simulink model "remoteMicrogrid"  (R2023a)
settings: Solver=FixedStepDiscrete  StartTime=0.0  StopTime=8  FixedStep=Ts  RelTol=1e-3
PreLoadFcn:
  | remoteMicrogridInputData
undefined symbols (not defined in the file): BESS, ControlRoom, DiscIntNeverNeededParam, Grid, Load, Machine, Microgrid, PV, T_on, Ts
libraries: ee_lib x46, eeGeneralControl x35, nesl_utility_internal x25, simulink x24, nesl_utility x20, fl_lib x17, slpidlib x12, eeTransforms x5, eeRmsMeasurement x4, eeTotalHarmonicDistorsion x4, eeSinusoidalMeasurement x3, batteryecm_lib x2
(part 4 of 5)

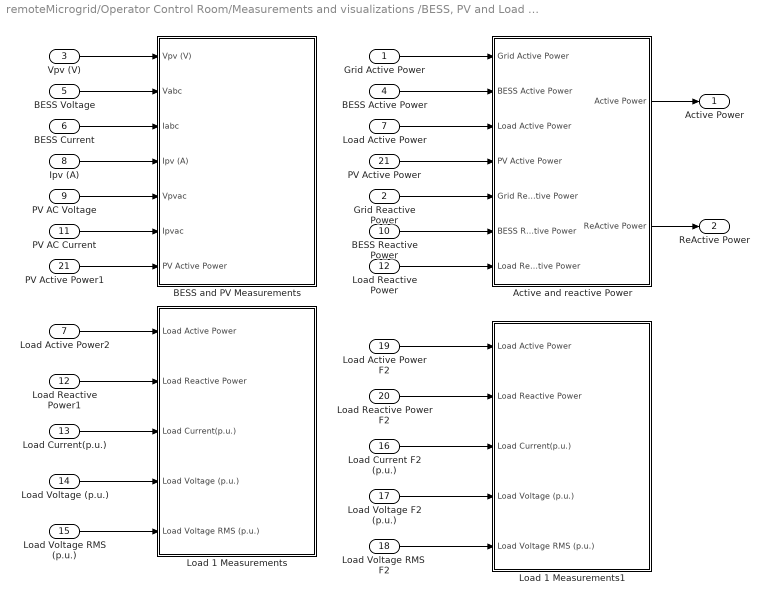
== system remoteMicrogrid/Operator Control Room/Measurements and visualizations /BESS, PV and Load Measurements ==
  Grid Active Power : Inport
  Grid Reactive Power : Inport  Port=2
  Vpv (V) : Inport  Port=3
  BESS Active Power : Inport  Port=4
  BESS Voltage : Inport  Port=5
  BESS Current : Inport  Port=6
  Load Active Power : Inport  Port=7
  Ipv (A) : Inport  Port=8
  PV AC Voltage : Inport  Port=9
  BESS Reactive Power : Inport  Port=10
  PV AC Current : Inport  Port=11
  Load Reactive Power : Inport  Port=12
  Load Current(p.u.) : Inport  Port=13
  Load Voltage (p.u.) : Inport  Port=14
  Load Voltage RMS (p.u.) : Inport  Port=15
  Load Current F2 (p.u.) : Inport  Port=16
  Load Voltage F2 (p.u.) : Inport  Port=17
  Load Voltage RMS  F2 : Inport  Port=18
  "Load Active Power F2 " : Inport  Port=19
  Load Reactive Power F2 : Inport  Port=20
  PV Active Power : Inport  Port=21
  Active and reactive Power : Subsystem
  BESS and PV Measurements : Subsystem
  Load 1 Measurements : Subsystem
  Load 1 Measurements1 : Subsystem
  Load Active Power2 : InportShadow  Port=7
  Load Reactive Power1 : InportShadow  Port=12
  PV Active Power1 : InportShadow  Port=21
  Active Power : Outport
  ReActive Power : Outport  Port=2
  wires:
  Vpv (V)/1 -> BESS and PV Measurements/1(Vpv (V))
  PV AC Current/1 -> BESS and PV Measurements/6(Ipvac)
  BESS Voltage/1 -> BESS and PV Measurements/2(Vabc)
  Load Reactive Power1/1 -> Load 1 Measurements/2(Load Reactive Power)
  PV AC Voltage/1 -> BESS and PV Measurements/5(Vpvac)
  Ipv (A)/1 -> BESS and PV Measurements/4(Ipv (A))
  BESS Current/1 -> BESS and PV Measurements/3(Iabc)
  BESS Reactive Power/1 -> Active and reactive Power/6(BESS Reactive Power)
  Load Voltage (p.u.)/1 -> Load 1 Measurements/4(Load Voltage (p.u.))
  Load Current(p.u.)/1 -> Load 1 Measurements/3(Load Current(p.u.))
  Load Active Power2/1 -> Load 1 Measurements/1(Load Active Power)
  Load Active Power/1 -> Active and reactive Power/3(Load Active Power)
  Load Voltage RMS (p.u.)/1 -> Load 1 Measurements/5(Load Voltage RMS (p.u.))
  Grid Active Power/1 -> Active and reactive Power/1(Grid Active Power)
  BESS Active Power/1 -> Active and reactive Power/2(BESS Active Power)
  Grid Reactive Power/1 -> Active and reactive Power/5(Grid Reactive Power)
  Load Reactive Power/1 -> Active and reactive Power/7(Load Reactive Power)
  "Load Active Power F2 "/1 -> Load 1 Measurements1/1(Load Active Power)
  Load Reactive Power F2/1 -> Load 1 Measurements1/2(Load Reactive Power)
  Load Current F2 (p.u.)/1 -> Load 1 Measurements1/3(Load Current(p.u.))
  Load Voltage F2 (p.u.)/1 -> Load 1 Measurements1/4(Load Voltage (p.u.))
  Load Voltage RMS  F2/1 -> Load 1 Measurements1/5(Load Voltage RMS (p.u.))
  PV Active Power/1 -> Active and reactive Power/4(PV Active Power)
  PV Active Power1/1 -> BESS and PV Measurements/7(PV Active Power)
  Active and reactive Power/1(Active Power) -> Active Power/1
  Active and reactive Power/2(ReActive Power) -> ReActive Power/1

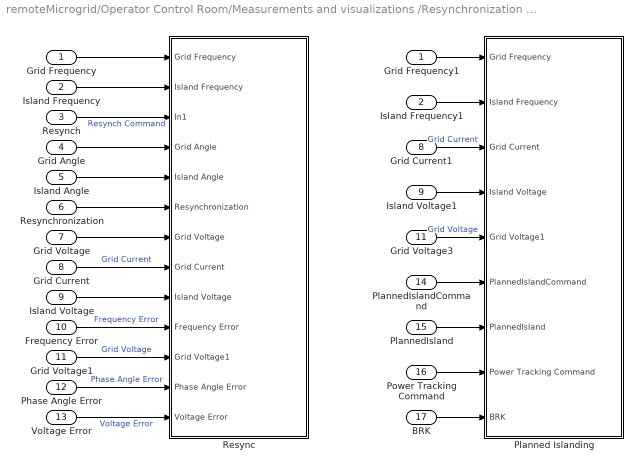
== system remoteMicrogrid/Operator Control Room/Measurements and visualizations /Resynchronization and Planned Islanding ==
  Grid Frequency : Inport
  Island Frequency : Inport  Port=2
  Resynch : Inport  Port=3
  Grid Angle : Inport  Port=4
  Island Angle : Inport  Port=5
  Resynchronization : Inport  Port=6
  Grid Voltage : Inport  Port=7
  Grid Current : Inport  Port=8
  Island Voltage : Inport  Port=9
  Frequency Error : Inport  Port=10
  Grid Voltage1 : Inport  Port=11
  Phase Angle Error : Inport  Port=12
  Voltage Error : Inport  Port=13
  PlannedIslandCommand : Inport  Port=14
  PlannedIsland : Inport  Port=15
  Power Tracking Command : Inport  Port=16
  BRK : Inport  Port=17
  Grid Current1 : InportShadow  Port=8
  Grid Frequency1 : InportShadow
  Grid Voltage3 : InportShadow  Port=11
  Island Frequency1 : InportShadow  Port=2
  Island Voltage1 : InportShadow  Port=9
  Planned Islanding : Subsystem
  Resync : Subsystem
  wires:
  Grid Frequency/1 -> Resync/1(Grid Frequency)
  Island Frequency/1 -> Resync/2(Island Frequency)
  Resynch/1 -> Resync/3(In1)  "Resynch Command"
  Grid Angle/1 -> Resync/4(Grid Angle)
  Island Angle/1 -> Resync/5(Island Angle)
  Resynchronization/1 -> Resync/6(Resynchronization)
  Grid Voltage/1 -> Resync/7(Grid Voltage)
  Grid Current/1 -> Resync/8(Grid Current)  "Grid Current"
  Island Voltage/1 -> Resync/9(Island Voltage)
  Frequency Error/1 -> Resync/10(Frequency Error)  "Frequency Error"
  Grid Voltage1/1 -> Resync/11(Grid Voltage1)  "Grid Voltage"
  Phase Angle Error/1 -> Resync/12(Phase Angle Error)  "Phase Angle Error"
  Voltage Error/1 -> Resync/13(Voltage Error)  "Voltage Error"
  Grid Frequency1/1 -> Planned Islanding/1(Grid Frequency)
  Island Frequency1/1 -> Planned Islanding/2(Island Frequency)
  Grid Current1/1 -> Planned Islanding/3(Grid Current)  "Grid Current"
  Island Voltage1/1 -> Planned Islanding/4(Island Voltage)
  Grid Voltage3/1 -> Planned Islanding/5(Grid Voltage1)  "Grid Voltage"
  PlannedIslandCommand/1 -> Planned Islanding/6(PlannedIslandCommand)
  PlannedIsland/1 -> Planned Islanding/7(PlannedIsland)
  Power Tracking Command/1 -> Planned Islanding/8(Power Tracking Command)
  BRK/1 -> Planned Islanding/9(BRK)

== system remoteMicrogrid/Operator Control Room/Monitoring of system performance/Load  ==
  In1 : Inport
  In2 : Inport  Port=2
  In3 : Inport  Port=3
  Constant1 : Constant  Value=0
  Constant2 : Constant  Value=0
  Constant3 : Constant  Value=0
  Gain : Gain  Gain=1/75
  Load Power and  Current MinMax : Scope  NumInputPorts=4
  Load Voltage MINMAX : Scope  NumInputPorts=4
  MinMax Running Resettable1 : simulink/Math Operations/MinMax Running Resettable  Function=min  vinit=1
  MinMax Running Resettable5 : simulink/Math Operations/MinMax Running Resettable  Function=max  vinit=1
  MinMax Running Resettable6 : simulink/Math Operations/MinMax Running Resettable  Function=min  vinit=0.707
  MinMax Running Resettable7 : simulink/Math Operations/MinMax Running Resettable  Function=max  vinit=0.707
  MinMax Running Resettable8 : simulink/Math Operations/MinMax Running Resettable  Function=min  vinit=0.707
  MinMax Running Resettable9 : simulink/Math Operations/MinMax Running Resettable  Function=max  vinit=0.491
  Subsystem4 : Subsystem
  start at 0.2 s2 : Subsystem
  start at 0.2 s4 : Subsystem
  start at 0.2 s5 : Subsystem
  wires:
  Constant2/1 -> MinMax Running Resettable7/2, MinMax Running Resettable6/2
  Constant1/1 -> MinMax Running Resettable1/2, MinMax Running Resettable5/2
  start at 0.2 s4/1(u) -> MinMax Running Resettable9/1, MinMax Running Resettable8/1
  MinMax Running Resettable7/1 -> Load Voltage MINMAX/4  "Load Voltage Max (pu)"
  Constant3/1 -> MinMax Running Resettable9/2, MinMax Running Resettable8/2
  MinMax Running Resettable8/1 -> Load Power and  Current MinMax/3  "Load Current Min (pu)"
  In1/1 -> start at 0.2 s2/1(In1)
  In2/1 -> start at 0.2 s4/1(In1)
  MinMax Running Resettable5/1 -> Load Power and  Current MinMax/2  "Load Power Max (pu)"
  In3/1 -> start at 0.2 s5/1(In1)
  Subsystem4/1(VoltageLow) -> Load Voltage MINMAX/1  "Load Voltage Crossed Low"
  start at 0.2 s2/1(u) -> MinMax Running Resettable7/1, MinMax Running Resettable6/1, Subsystem4/1(Voltage)
  Gain/1 -> MinMax Running Resettable5/1, MinMax Running Resettable1/1
  MinMax Running Resettable9/1 -> Load Power and  Current MinMax/4  "Load Current Max (pu)"
  start at 0.2 s5/1(u) -> Gain/1
  Subsystem4/2(VoltageHigh) -> Load Voltage MINMAX/2  "Load Voltage Crossed High"
  MinMax Running Resettable6/1 -> Load Voltage MINMAX/3  "Load Voltage Min (pu)"
  MinMax Running Resettable1/1 -> Load Power and  Current MinMax/1  "Load Power Min (pu)"

== system remoteMicrogrid/Operator Control Room/Monitoring of system performance/Microgrid ==
  In1 : Inport
  In2 : Inport  Port=2
  Constant : Constant  Value=0
  Constant4 : Constant  Value=0
  Island Frequency MINMAX : Scope  NumInputPorts=4
  Island Voltage MINMAX : Scope  NumInputPorts=4
  Low-Pass Filter (Discrete or Continuous) : eeGeneralControl/Low-Pass Filter (Discrete or Continuous)  K=1  T=0.04  B=inf  A=-inf  init_option=Inherited from block input  x0=0  Ts=Ts
  Low-Pass Filter (Discrete or Continuous)1 : eeGeneralControl/Low-Pass Filter (Discrete or Continuous)  K=1  T=0.04  B=inf  A=-inf  init_option=Inherited from block input  x0=0  Ts=Ts
  MinMax Running Resettable : simulink/Math Operations/MinMax Running Resettable  Function=max  vinit=Grid.Frequency
  MinMax Running Resettable2 : simulink/Math Operations/MinMax Running Resettable  Function=max  vinit=1
  MinMax Running Resettable3 : simulink/Math Operations/MinMax Running Resettable  Function=min  vinit=1
  MinMax Running Resettable4 : simulink/Math Operations/MinMax Running Resettable  Function=min  vinit=Grid.Frequency
  Subsystem : Subsystem
  Subsystem3 : Subsystem
  start at 2 s : Subsystem
  start at 2 s1 : Subsystem
  wires:
  Subsystem/1(FrequencyLow) -> Island Frequency MINMAX/1  "Microgrid Frequency Croosed Low (59 HZ)"
  Constant/1 -> MinMax Running Resettable4/2, MinMax Running Resettable/2
  In1/1 -> Low-Pass Filter (Discrete or Continuous)/1
  Subsystem3/1(VoltageLow) -> Island Voltage MINMAX/1  "Microgrid Voltage Crossed Low (0.95 pu)"
  Subsystem/2(FrequencyHigh) -> Island Frequency MINMAX/2  "Microgrid Frequency Crossed High (62 Hz)"
  In2/1 -> Low-Pass Filter (Discrete or Continuous)1/1
  MinMax Running Resettable2/1 -> Island Voltage MINMAX/3  "Microgrid Voltage Max (pu)"
  start at 2 s/1(u) -> MinMax Running Resettable4/1, MinMax Running Resettable/1, Subsystem/1(Frequency)
  Subsystem3/2(VoltageHigh) -> Island Voltage MINMAX/2  "Microgrid Voltage Crossed High (1.1 pu)"
  start at 2 s1/1(u) -> MinMax Running Resettable3/1, MinMax Running Resettable2/1, Subsystem3/1(Voltage)
  Constant4/1 -> MinMax Running Resettable3/2, MinMax Running Resettable2/2
  MinMax Running Resettable4/1 -> Island Frequency MINMAX/4  "Microgrid Frequency Min (Hz)"
  MinMax Running Resettable3/1 -> Island Voltage MINMAX/4  "Microgrid Voltage Min (pu)"
  MinMax Running Resettable/1 -> Island Frequency MINMAX/3  "Microgrid Frequency Max (Hz)"
  Low-Pass Filter (Discrete or Continuous)/1 -> start at 2 s/1(In1)
  Low-Pass Filter (Discrete or Continuous)1/1 -> start at 2 s1/1(In1)

== system remoteMicrogrid/Operator Control Room/Monitoring of system performance/Subsystem ==
  Active and Reactive Power : Inport
  mLoadF2 : Inport  Port=2
  Bus Selector : BusSelector  OutputSignals=signal1.Grid Active Power,signal1.BESS Active Power,signal1.Load Active Power,signal1.PV Active Power),signal2.Grid Reactive Power,signal2.BESS Reactive Power,signal2.Load Reactive Power
  Bus Selector1 : BusSelector  OutputSignals=reactive powerF2
  Bus Selector2 : BusSelector  OutputSignals=active powerF2
  Constant4 : Constant  Value=0
  MinMax Running Resettable1 : simulink/Math Operations/MinMax Running Resettable  Function=max  vinit=1
  MinMax Running Resettable2 : simulink/Math Operations/MinMax Running Resettable  Function=max  vinit=1
  Sum : Sum  Inputs=-++-+
  Sum1 : Sum  Inputs=++--
  Terminator : Terminator
  Terminator1 : Terminator
  mLoadF1 : InportShadow  Port=2
  start at 2.5 s : Subsystem
  start at 2.5 s1 : Subsystem
  wires:
  start at 2.5 s1/1(u) -> MinMax Running Resettable2/1
  Constant4/1 -> MinMax Running Resettable1/2, MinMax Running Resettable2/2
  Bus Selector/5 -> Sum1/1  "<Grid Reactive Power>"
  Sum/1 -> start at 2.5 s1/1(ActivePower)
  Sum1/1 -> start at 2.5 s/1(ReactivePower)
  Bus Selector/7 -> Sum1/3  "<Load Reactive Power>"
  Bus Selector/6 -> Sum1/2  "<BESS Reactive Power>"
  Active and Reactive Power/1 -> Bus Selector/1
  MinMax Running Resettable2/1 -> Terminator/1  "Max Active Power Loss (kW)"
  start at 2.5 s/1(u) -> MinMax Running Resettable1/1
  MinMax Running Resettable1/1 -> Terminator1/1  "Max Active Power Loss (kW)"
  mLoadF2/1 -> Bus Selector1/1
  Bus Selector1/1 -> Sum1/4  "<reactive powerF2>"
  mLoadF1/1 -> Bus Selector2/1
  Bus Selector/4 -> Sum/5  "<PV Active Power)>"
  Bus Selector/3 -> Sum/4  "<Load Active Power>"
  Bus Selector/2 -> Sum/3  "<BESS Active Power>"
  Bus Selector/1 -> Sum/2  "<Grid Active Power>"
  Bus Selector2/1 -> Sum/1  "<active powerF2>"

== system remoteMicrogrid/Operator Control Room/Monitoring of system performance/THD ==
  mLoad : Inport
  In2 : Inport  Port=2
  MGController : Inport  Port=3
  In4 : Inport  Port=4
  THD : Scope  NumInputPorts=4
  Total Harmonic Distortion{,1..3} (4 alike) : eeTotalHarmonicDistorsion/Total Harmonic Distortion  f=60  Ts=Ts
  wires:
  Total Harmonic Distortion1/1 -> THD/2  "Load Current THD (%)"
  Total Harmonic Distortion3/1 -> THD/4  "PCC Current THD (%)"
  Total Harmonic Distortion2/1 -> THD/3  "PCC Voltage THD (%)"
  Total Harmonic Distortion/1 -> THD/1  "Load Voltage THD (%)"
  In2/1 -> Total Harmonic Distortion1/1
  mLoad/1 -> Total Harmonic Distortion/1
  MGController/1 -> Total Harmonic Distortion2/1
  In4/1 -> Total Harmonic Distortion3/1

== system remoteMicrogrid/PV /30 kW PV/L Filter1 ==
  RLC (Three-Phase) : ee_lib/Passive/RLC Assemblies/RLC (Three-Phase)  component_structure=ee.enum.rlc.structure.L  R=1e-3 Ohm  L=PV.L H  C=1e-6 F  R_parasitic=0 Ohm  G_parasitic=0 1/Ohm  IL_specify=off  IL_priority=High  IL=[0, 0, 0] A  IL_nominal_specify=off  IL_nominal_unit=A  IL_nominal_value=1  VC_specify=off  VC_priority=High  VC=[0, 0, 0] V  VC_nominal_specify=off  VC_nominal_unit=V  VC_nominal_value=1
      settings: InternalSimscapePortConfiguration="{\"Bottom\":[],\"Left\":[{\"id\":\"N1\",\"label\":\"~1\",\"type\":\"foundation.electrical.three_phase\"}],\"Right\":[{\"id\":\"N2\",\"label\":\"~2\",\"type\":\"foundation.electrical.three_phase\"}],\"Top\":[]}"
  " ~ " : PMIOPort  Side=Right
  ~ : PMIOPort  Port=2  Side=Left
  connections:
  " ~ "/RConn1 -- RLC (Three-Phase)/RConn1
  RLC (Three-Phase)/LConn1 -- ~/RConn1

== system remoteMicrogrid/PV /30 kW PV/Measurement1 ==
  u : Inport
  Lead-Lag (Discrete or Continuous) : eeGeneralControl/Lead-Lag (Discrete or Continuous)  T1=0  T2=PV.t_sensor  B=inf  A=-inf  init_option=Inherited from block input  x0=0  Ts=Ts
      settings: LibrarySourceBlock=|
      | ee_sl_lib/General Control/Lead-Lag
      | (Discrete or Continuous)
  Out Bus Element : Outport  PortName=ipv1  Element=1
  wires:
  Lead-Lag (Discrete or Continuous)/1 -> Out Bus Element/1
  u/1 -> Lead-Lag (Discrete or Continuous)/1

== system remoteMicrogrid/PV /30 kW PV/PV Inverter 2 ==
  In Bus Element : Inport  PortName=PV
  In Bus Element1 : Inport  Port=2  PortName=ipv1
  Constant : Constant  Value=1000  SampleTime=-1
  PV Control : Subsystem
  PV Plant : Subsystem
  Conn1 : PMIOPort  Side=Right
  PV power : Outport
  wires:
  Constant/1 -> PV Plant/1(Insolation)
  [m] -> PV Plant/2(mod)
  PV Plant/1(PV_plant1) -> PV Control/1(PV_plant1)
  PV Control/1(mabc) -> [m]
  In Bus Element/1 -> PV Control/2(PV)
  In Bus Element1/1 -> PV Control/3(ipv1)
  PV Control/2(PV power) -> PV power/1
  connections:
  Conn1/RConn1 -- PV Plant/RConn1

== system remoteMicrogrid/PV /PLL & Measurements/Measurement2 ==
  u : Inport
  Lead-Lag (Discrete or Continuous) : eeGeneralControl/Lead-Lag (Discrete or Continuous)  T1=0  T2=PV.t_sensor  B=inf  A=-inf  init_option=Inherited from block input  x0=0  Ts=Ts
      settings: LibrarySourceBlock=|
      | ee_sl_lib/General Control/Lead-Lag
      | (Discrete or Continuous)
  Vg : Outport
  wires:
  Lead-Lag (Discrete or Continuous)/1 -> Vg/1
  u/1 -> Lead-Lag (Discrete or Continuous)/1

== system remoteMicrogrid/PV /PLL & Measurements/Subsystem ==
  abc : Inport
  Demux : Demux  Outputs=3
  Park Transform : eeTransforms/Park Transform  AxisAlignment=Q-axis  PowerInvariant=off
  "Sinusoidal Measurement (PLL, Three-Phase)1" : eeSinusoidalMeasurementV2/Sinusoidal Measurement (PLL, Three-Phase)  Kp_LF=PV.Kp_pll  Ki_LF=PV.Ki_pll  F0=Grid.Frequency  Theta0=0  Ts=-1
      settings: LibrarySourceBlock=|
      | ee_sl_lib/Measurements/Sinusoidal Measurement
      | (PLL, Three-Phase)
  Terminator : Terminator
  mag : Outport
  freq : Outport  Port=2
  angle : Outport  Port=3
  Vd : Outport  Port=4
  Vq : Outport  Port=5
  wires:
  Demux/3 -> Terminator/1
  abc/1 -> "Sinusoidal Measurement (PLL, Three-Phase)1"/1, Park Transform/1
  Park Transform/1 -> Demux/1
  Demux/1 -> Vd/1
  Demux/2 -> Vq/1
  "Sinusoidal Measurement (PLL, Three-Phase)1"/2 -> Park Transform/2, angle/1
  "Sinusoidal Measurement (PLL, Three-Phase)1"/1 -> freq/1
  "Sinusoidal Measurement (PLL, Three-Phase)1"/3 -> mag/1

== system remoteMicrogrid/Diesel Substation, BESS, & Microgrid Controller/BESS and Controller/BESS Control/Inverter Active & Reactive Power  ==
  Vabc : Inport
  Iabc : Inport  Port=2
  Demux : Demux  Outputs=3
  Gain : Gain  Gain=1/sqrt(3)
  Minus : Sum  Inputs=+-
  Minus1 : Sum  Inputs=+-
  Minus2 : Sum  Inputs=+-
  Mux : Mux  Inputs=3
  Product : Product
  Product1 : Product
  Sum of Elements : Sum  Inputs=+
  Sum of Elements1 : Sum  Inputs=+
  P : Outport  VectorParamsAs1DForOutWhenUnconnected=off
  Q : Outport  Port=2  VectorParamsAs1DForOutWhenUnconnected=off
  wires:
  Minus/1 -> Mux/3
  Minus2/1 -> Mux/2
  Minus1/1 -> Mux/1
  Sum of Elements1/1 -> Gain/1
  Product1/1 -> Sum of Elements1/1
  Mux/1 -> Product1/2
  Demux/3 -> Minus1/2, Minus2/1
  Demux/2 -> Minus/2, Minus1/1
  Demux/1 -> Minus/1, Minus2/2
  Product/1 -> Sum of Elements/1
  Iabc/1 -> Product/2, Product1/1
  Vabc/1 -> Product/1, Demux/1
  Sum of Elements/1 -> P/1
  Gain/1 -> Q/1

== system remoteMicrogrid/Diesel Substation, BESS, & Microgrid Controller/Diesel Generator/Governor and Prime Mover /Governor ==
  pu_velocity : Inport
  1/T_G : Gain  Gain=1/T_G
  1/droop : Gain  Gain=1/(droop_percentage/100)
  Delta load setpoint : Sum  Inputs=+-|
  Delta speed : Sum  Inputs=-+|
  Discrete-Time Integrator1 : DiscreteIntegrator  InitialCondition=pu_torque0  SampleTime=-1  ICPrevOutput=DiscIntNeverNeededParam  ICPrevScaledInput=DiscIntNeverNeededParam
  Load_setpoint : Constant  Value=pu_load_reference_setpoint
  Speed_ref : Constant  Value=pu_speed_reference
  Subtract : Sum  Inputs=|+-
  delta_y : Outport  VectorParamsAs1DForOutWhenUnconnected=off
  wires:
  Speed_ref/1 -> Delta speed/1
  Delta speed/1 -> 1/droop/1
  Load_setpoint/1 -> Delta load setpoint/1
  pu_velocity/1 -> Delta speed/2
  1/droop/1 -> Delta load setpoint/2
  Delta load setpoint/1 -> Subtract/1
  Subtract/1 -> 1/T_G/1
  1/T_G/1 -> Discrete-Time Integrator1/1
  Discrete-Time Integrator1/1 -> delta_y/1, Subtract/2

== system remoteMicrogrid/Diesel Substation, BESS, & Microgrid Controller/Diesel Generator/Governor and Prime Mover /Non-reheat turbine ==
  delta_y : Inport
  1/T_CH : Gain  Gain=1/T_CH
  Discrete-Time Integrator1 : DiscreteIntegrator  InitialCondition=pu_torque0  SampleTime=-1  ICPrevOutput=DiscIntNeverNeededParam  ICPrevScaledInput=DiscIntNeverNeededParam
  Sum : Sum  Inputs=|+-
  torque : Outport  VectorParamsAs1DForOutWhenUnconnected=off
  wires:
  delta_y/1 -> Sum/1
  Sum/1 -> 1/T_CH/1
  1/T_CH/1 -> Discrete-Time Integrator1/1
  Discrete-Time Integrator1/1 -> Sum/2, torque/1

== system remoteMicrogrid/Diesel Substation, BESS, & Microgrid Controller/Microgrid Controller/PLL/PLL ==
  abc : Inport
  "Sinusoidal Measurement (PLL, Three-Phase)" : eeSinusoidalMeasurement/Sinusoidal Measurement (PLL, Three-Phase)  Kp_LF=Grid.PLL_Kp  Ki_LF=Grid.PLL_Ki  F0=Grid.Frequency  Theta0=0  Ts=Ts
  Subsystem : Subsystem
  start at 0.25 s : Subsystem
  start at 0.25 s1 : Subsystem
  fre : Outport
  angle : Outport  Port=2
  mag : Outport  Port=3
  wires:
  abc/1 -> "Sinusoidal Measurement (PLL, Three-Phase)"/1
  "Sinusoidal Measurement (PLL, Three-Phase)"/3 -> start at 0.25 s1/1(In1)
  "Sinusoidal Measurement (PLL, Three-Phase)"/2 -> Subsystem/1(In)
  Subsystem/1(Out) -> angle/1
  "Sinusoidal Measurement (PLL, Three-Phase)"/1 -> start at 0.25 s/1(In1)
  start at 0.25 s1/1(u) -> mag/1
  start at 0.25 s/1(u) -> fre/1

== system remoteMicrogrid/Diesel Substation, BESS, & Microgrid Controller/Microgrid Controller/PLL/PLL start at 0.2 s ==
  PCC measurement : Inport
  Constant : Constant  Value=0
  Step : Step  Time=0.2  SampleTime=Ts
  Switch : Switch  Criteria=u2 > Threshold  Threshold=0.5  SaturateOnIntegerOverflow=off  InputSameDT=off
  mPLL : Outport
  wires:
  PCC measurement/1 -> Switch/1
  Switch/1 -> mPLL/1
  Constant/1 -> Switch/3
  Step/1 -> Switch/2

== system remoteMicrogrid/Diesel Substation, BESS, & Microgrid Controller/Microgrid Controller/PLL/PLL starts at 0.2 s ==
  PCC measurement : Inport
  Constant1 : Constant  Value=0
  Step : Step  Time=0.2  SampleTime=Ts
  Switch : Switch  Criteria=u2 > Threshold  Threshold=0.5  SaturateOnIntegerOverflow=off  InputSameDT=off
  mPLL : Outport
  wires:
  PCC measurement/1 -> Switch/1
  Constant1/1 -> Switch/3
  Switch/1 -> mPLL/1
  Step/1 -> Switch/2

== system remoteMicrogrid/Diesel Substation, BESS, & Microgrid Controller/Microgrid Controller/PLL/PLL1 ==
  abc : Inport
  "Sinusoidal Measurement (PLL, Three-Phase)" : eeSinusoidalMeasurement/Sinusoidal Measurement (PLL, Three-Phase)  Kp_LF=Grid.PLL_Kp  Ki_LF=Grid.PLL_Ki  F0=Grid.Frequency  Theta0=0  Ts=Ts
  Subsystem : Subsystem
  start at 0.25 s : Subsystem
  start at 0.25 s2 : Subsystem
  fre : Outport
  angle : Outport  Port=2
  mag : Outport  Port=3
  wires:
  "Sinusoidal Measurement (PLL, Three-Phase)"/1 -> start at 0.25 s2/1(In1)
  Subsystem/1(Out) -> angle/1
  "Sinusoidal Measurement (PLL, Three-Phase)"/2 -> Subsystem/1(In)
  "Sinusoidal Measurement (PLL, Three-Phase)"/3 -> start at 0.25 s/1(In1)
  abc/1 -> "Sinusoidal Measurement (PLL, Three-Phase)"/1
  start at 0.25 s/1(u) -> mag/1
  start at 0.25 s2/1(u) -> fre/1

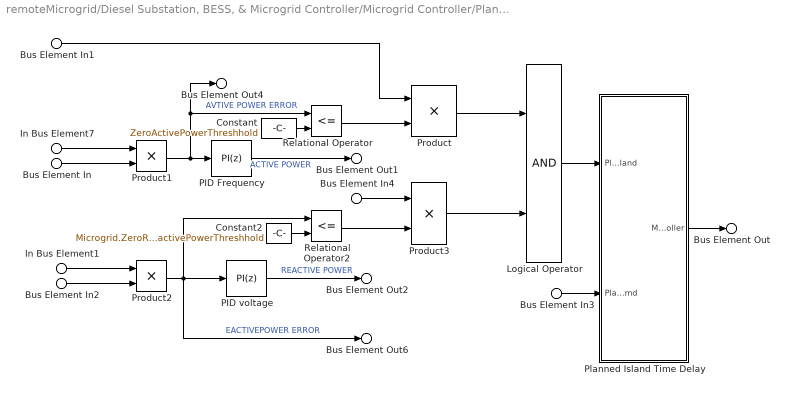
== system remoteMicrogrid/Diesel Substation, BESS, & Microgrid Controller/Microgrid Controller/Planned Island from Diesel/Control for Zero Powerflow for planned island ==
  Bus Element In{,1..4} (5 alike) : Inport  PortName=ControlRoomSubstation  Element=PlannedIslandCmd
  In Bus Element1 : Inport  Port=2  PortName=mPCCPLL  Element=PCC.mPCC.reactivepower
  In Bus Element7 : Inport  Port=2  PortName=mPCCPLL  Element=PCC.mPCC.activepower
  Constant : Constant  Value=ZeroActivePowerThreshhold  SampleTime=-1
  Constant2 : Constant  Value=Microgrid.ZeroReactivePowerThreshhold
  Logical Operator : Logic  AllPortsSameDT=off  OutDataTypeStr=boolean
  PID Frequency : slpidlib/PID Controller  Controller=PI  Form=Parallel  TimeDomain=Discrete-time  UseExternalTs=off  SampleTime=Ts  IntegratorMethod=Forward Euler  FilterMethod=Forward Euler  ControllerParametersSource=internal  P=KP_P_plannedisland  I=KI_P_plannedisland  UseKiTs=off  D=0  N=100  UseFilter=on  TunerSelectOption=Frequency Response Based  InitialConditionSource=internal  InitialConditionForIntegrator=0  InitialConditionForFilter=0  DifferentiatorICPrevScaledInput=0  ExternalReset=none  TrackingMode=off  Kt=1  LimitOutput=off  SatLimitsSource=internal  UpperSaturationLimit=0.05  LowerSaturationLimit=-0.05  LinearizeAsGain=on  AntiWindupMode=clamping  Kb=1  LimitIntegrator=off  UpperIntegratorSaturationLimit=inf  LowerIntegratorSaturationLimit=-inf  POutMin=[]  POutMax=[]  IOutMin=[]  IOutMax=[]  DOutMin=[]  DOutMax=[]  NOutMin=[]  NOutMax=[]  SumOutMin=[]  SumOutMax=[]  SaturationOutMin=[]  SaturationOutMax=[]  PParamMin=[]  PParamMax=[]  IParamMin=[]  IParamMax=[]  DParamMin=[]  DParamMax=[]  NParamMin=[]  NParamMax=[]  KbParamMin=[]  KbParamMax=[]  KtParamMin=[]  KtParamMax=[]  KbOutMin=[]  KbOutMax=[]  KtOutMin=[]  KtOutMax=[]  IntegratorOutMin=[]  IntegratorOutMax=[]  FilterOutMin=[]  FilterOutMax=[]  SumI1OutMin=[]  SumI1OutMax=[]  SumI2OutMin=[]  SumI2OutMax=[]  SumI3OutMin=[]  SumI3OutMax=[]  SumI4OutMin=[]  SumI4OutMax=[]  SumDOutMin=[]  SumDOutMax=[]  DifferentiatorOutMin=[]  DifferentiatorOutMax=[]  FilterDiffOutCoefMin=[]  FilterDiffOutCoefMax=[]  ReciprocalOutMin=[]  ReciprocalOutMax=[]  SumDenOutMin=[]  SumDenOutMax=[]  SumNumOutMin=[]  SumNumOutMax=[]  DivideOutMin=[]  DivideOutMax=[]  UdiffTsProdOutMin=[]  UdiffTsProdOutMax=[]  NTsProdOutMin=[]  NTsProdOutMax=[]  UintegralTsProdOutMin=[]  UintegralTsProdOutMax=[]  UngainTsProdOutMin=[]  UngainTsProdOutMax=[]  ClampingZeroOutDataTypeStr=Inherit: Inherit via back propagation  ClampingZeroOutMin=[]  ClampingZeroOutMax=[]  FilterDenConstantOutDataTypeStr=Inherit: Inherit via back propagation  FilterDenConstantOutMin=[]  FilterDenConstantOutMax=[]  PCopyOutDataTypeStr=Inherit: Inherit via back propagation  PCopyOutMin=[]  PCopyOutMax=[]  NCopyOutDataTypeStr=Inherit: Inherit via back propagation  NCopyOutMin=[]  NCopyOutMax=[]  IntegratorContinuousStateAttributes=''  IntegratorStateMustResolveToSignalObject=off  IntegratorRTWStateStorageClass=Auto  FilterContinuousStateAttributes=''  FilterStateMustResolveToSignalObject=off  FilterRTWStateStorageClass=Auto  ParallelPVariant=InternalParameters  IdealPVariant=Disabled  IVariant=InternalParameters  DVariant=Disabled  IntegratorVariant=Discrete  SatVariant=Disabled  AWVariant=Passthrough  PCopyVariant=Disabled  TRVariant=Disabled  FdbkBlocksVariant=Forward  IdealPFdbkVariant=Disabled  SatFdbkVariant=Disabled  DerivativeFilterVariant=Disabled  NVariant=Disabled  NCopyVariant=Disabled_SignalSpec  FilterICVariant=Disabled  IntegratorICVariant=InternalICs  ExternalResetVariant=Disabled  TRSumVariant=Passthrough  SumFdbkVariant=Disabled  SumVariant=Sum_PI  TsampFilterVariant=InternalTs  TsampNgainVariant=Passthrough  TsampIntegralVariant=Disabled_SignalSpec  ExternalSaturationOutDataTypeStr=Inherit: Same as second input
  PID voltage : slpidlib/PID Controller  Controller=PI  Form=Parallel  TimeDomain=Discrete-time  UseExternalTs=off  SampleTime=Ts  IntegratorMethod=Forward Euler  FilterMethod=Forward Euler  ControllerParametersSource=internal  P=Microgrid.KP_Q_plannedisland  I=Microgrid.KI_Q_plannedisland  UseKiTs=off  D=0  N=100  UseFilter=on  TunerSelectOption=Frequency Response Based  InitialConditionSource=internal  InitialConditionForIntegrator=0  InitialConditionForFilter=0  DifferentiatorICPrevScaledInput=0  ExternalReset=none  TrackingMode=off  Kt=1  LimitOutput=off  SatLimitsSource=internal  UpperSaturationLimit=0.05  LowerSaturationLimit=-0.05  LinearizeAsGain=on  AntiWindupMode=clamping  Kb=1  LimitIntegrator=off  UpperIntegratorSaturationLimit=inf  LowerIntegratorSaturationLimit=-inf  POutMin=[]  POutMax=[]  IOutMin=[]  IOutMax=[]  DOutMin=[]  DOutMax=[]  NOutMin=[]  NOutMax=[]  SumOutMin=[]  SumOutMax=[]  SaturationOutMin=[]  SaturationOutMax=[]  PParamMin=[]  PParamMax=[]  IParamMin=[]  IParamMax=[]  DParamMin=[]  DParamMax=[]  NParamMin=[]  NParamMax=[]  KbParamMin=[]  KbParamMax=[]  KtParamMin=[]  KtParamMax=[]  KbOutMin=[]  KbOutMax=[]  KtOutMin=[]  KtOutMax=[]  IntegratorOutMin=[]  IntegratorOutMax=[]  FilterOutMin=[]  FilterOutMax=[]  SumI1OutMin=[]  SumI1OutMax=[]  SumI2OutMin=[]  SumI2OutMax=[]  SumI3OutMin=[]  SumI3OutMax=[]  SumI4OutMin=[]  SumI4OutMax=[]  SumDOutMin=[]  SumDOutMax=[]  DifferentiatorOutMin=[]  DifferentiatorOutMax=[]  FilterDiffOutCoefMin=[]  FilterDiffOutCoefMax=[]  ReciprocalOutMin=[]  ReciprocalOutMax=[]  SumDenOutMin=[]  SumDenOutMax=[]  SumNumOutMin=[]  SumNumOutMax=[]  DivideOutMin=[]  DivideOutMax=[]  UdiffTsProdOutMin=[]  UdiffTsProdOutMax=[]  NTsProdOutMin=[]  NTsProdOutMax=[]  UintegralTsProdOutMin=[]  UintegralTsProdOutMax=[]  UngainTsProdOutMin=[]  UngainTsProdOutMax=[]  ClampingZeroOutDataTypeStr=Inherit: Inherit via back propagation  ClampingZeroOutMin=[]  ClampingZeroOutMax=[]  FilterDenConstantOutDataTypeStr=Inherit: Inherit via back propagation  FilterDenConstantOutMin=[]  FilterDenConstantOutMax=[]  PCopyOutDataTypeStr=Inherit: Inherit via back propagation  PCopyOutMin=[]  PCopyOutMax=[]  NCopyOutDataTypeStr=Inherit: Inherit via back propagation  NCopyOutMin=[]  NCopyOutMax=[]  IntegratorContinuousStateAttributes=''  IntegratorStateMustResolveToSignalObject=off  IntegratorRTWStateStorageClass=Auto  FilterContinuousStateAttributes=''  FilterStateMustResolveToSignalObject=off  FilterRTWStateStorageClass=Auto  ParallelPVariant=InternalParameters  IdealPVariant=Disabled  IVariant=InternalParameters  DVariant=Disabled  IntegratorVariant=Discrete  SatVariant=Disabled  AWVariant=Passthrough  PCopyVariant=Disabled  TRVariant=Disabled  FdbkBlocksVariant=Forward  IdealPFdbkVariant=Disabled  SatFdbkVariant=Disabled  DerivativeFilterVariant=Disabled  NVariant=Disabled  NCopyVariant=Disabled_SignalSpec  FilterICVariant=Disabled  IntegratorICVariant=InternalICs  ExternalResetVariant=Disabled  TRSumVariant=Passthrough  SumFdbkVariant=Disabled  SumVariant=Sum_PI  TsampFilterVariant=InternalTs  TsampNgainVariant=Passthrough  TsampIntegralVariant=Disabled_SignalSpec  ExternalSaturationOutDataTypeStr=Inherit: Same as second input
  Planned Island Time Delay : Subsystem
  Product{,1..3} (4 alike) : Product
  Relational Operator : RelationalOperator  Operator=<=  OutDataTypeStr=boolean  RndMeth=Simplest  InputSameDT=off
  Relational Operator2 : RelationalOperator  Operator=<=  OutDataTypeStr=boolean  RndMeth=Simplest  InputSameDT=off
  Bus Element Out : Outport  PortName=MGController  Element=plannedisland
  Bus Element Out1 : Outport  PortName=MGController  Element=plannedislandP
  Bus Element Out2 : Outport  PortName=MGController  Element=plannedislandQ
  Bus Element Out4 : Outport  PortName=MGController  Element=activepowererror
  Bus Element Out6 : Outport  PortName=MGController  Element=reactivepowerrror
  wires:
  Logical Operator/1 -> Planned Island Time Delay/1(PlannedIsland)
  Planned Island Time Delay/1(MGController) -> Bus Element Out/1
  Bus Element In3/1 -> Planned Island Time Delay/2(PlannedislandCmd)
  PID voltage/1 -> Bus Element Out2/1  "REACTIVE POWER"
  Bus Element In2/1 -> Product2/2
  Bus Element In/1 -> Product1/2
  Product2/1 -> PID voltage/1, Bus Element Out6/1, Relational Operator2/1  "EACTIVEPOWER ERROR"
  Product1/1 -> PID Frequency/1, Relational Operator/1, Bus Element Out4/1  "AVTIVE POWER ERROR"
  PID Frequency/1 -> Bus Element Out1/1  "ACTIVE POWER"
  Constant2/1 -> Relational Operator2/2
  Constant/1 -> Relational Operator/2
  In Bus Element1/1 -> Product2/1
  In Bus Element7/1 -> Product1/1
  Bus Element In1/1 -> Product/1
  Relational Operator/1 -> Product/2
  Product/1 -> Logical Operator/1
  Product3/1 -> Logical Operator/2
  Relational Operator2/1 -> Product3/2
  Bus Element In4/1 -> Product3/1

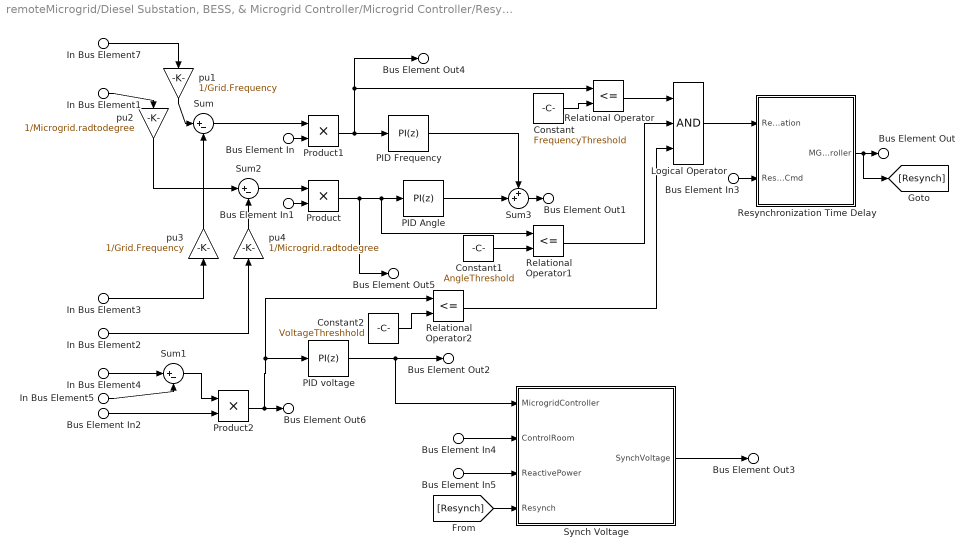
== system remoteMicrogrid/Diesel Substation, BESS, & Microgrid Controller/Microgrid Controller/Resynchronization to Diesel/Frequency and voltage matching ==
  Bus Element In5 : Inport  PortName=BESS  Element=reactive power
  Bus Element In{,1..4} (5 alike) : Inport  Port=2  PortName=ControlRoomSubstation  Element=ResynchCmd
  In Bus Element7 : Inport  Port=3  PortName=mPCCPLL  Element=Grid.frequency
  In Bus Element1 : Inport  Port=3  PortName=mPCCPLL  Element=Grid.angle
  In Bus Element4 : Inport  Port=3  PortName=mPCCPLL  Element=Grid.voltage
  In Bus Element3 : Inport  Port=3  PortName=mPCCPLL  Element=Island.frequency
  In Bus Element2 : Inport  Port=3  PortName=mPCCPLL  Element=Island.angle
  In Bus Element5 : Inport  Port=3  PortName=mPCCPLL  Element=Island.voltage
  Constant : Constant  Value=FrequencyThreshold  SampleTime=-1
  Constant1 : Constant  Value=AngleThreshold
  Constant2 : Constant  Value=VoltageThreshhold
  Logical Operator : Logic  Inputs=3  AllPortsSameDT=off  OutDataTypeStr=boolean
  PID Angle : slpidlib/PID Controller  Controller=PI  Form=Parallel  TimeDomain=Discrete-time  UseExternalTs=off  SampleTime=2*Ts  IntegratorMethod=Forward Euler  FilterMethod=Forward Euler  ControllerParametersSource=internal  P=Microgrid.KP_Ang_resynch  I=Microgrid.KI_Ang_resynch  UseKiTs=off  D=0  N=100  UseFilter=on  TunerSelectOption=Frequency Response Based  InitialConditionSource=internal  InitialConditionForIntegrator=0  InitialConditionForFilter=0  DifferentiatorICPrevScaledInput=0  ExternalReset=none  TrackingMode=off  Kt=1  LimitOutput=off  SatLimitsSource=internal  UpperSaturationLimit=0.05  LowerSaturationLimit=-0.05  LinearizeAsGain=on  AntiWindupMode=clamping  Kb=1  LimitIntegrator=off  UpperIntegratorSaturationLimit=inf  LowerIntegratorSaturationLimit=-inf  POutMin=[]  POutMax=[]  IOutMin=[]  IOutMax=[]  DOutMin=[]  DOutMax=[]  NOutMin=[]  NOutMax=[]  SumOutMin=[]  SumOutMax=[]  SaturationOutMin=[]  SaturationOutMax=[]  PParamMin=[]  PParamMax=[]  IParamMin=[]  IParamMax=[]  DParamMin=[]  DParamMax=[]  NParamMin=[]  NParamMax=[]  KbParamMin=[]  KbParamMax=[]  KtParamMin=[]  KtParamMax=[]  KbOutMin=[]  KbOutMax=[]  KtOutMin=[]  KtOutMax=[]  IntegratorOutMin=[]  IntegratorOutMax=[]  FilterOutMin=[]  FilterOutMax=[]  SumI1OutMin=[]  SumI1OutMax=[]  SumI2OutMin=[]  SumI2OutMax=[]  SumI3OutMin=[]  SumI3OutMax=[]  SumI4OutMin=[]  SumI4OutMax=[]  SumDOutMin=[]  SumDOutMax=[]  DifferentiatorOutMin=[]  DifferentiatorOutMax=[]  FilterDiffOutCoefMin=[]  FilterDiffOutCoefMax=[]  ReciprocalOutMin=[]  ReciprocalOutMax=[]  SumDenOutMin=[]  SumDenOutMax=[]  SumNumOutMin=[]  SumNumOutMax=[]  DivideOutMin=[]  DivideOutMax=[]  UdiffTsProdOutMin=[]  UdiffTsProdOutMax=[]  NTsProdOutMin=[]  NTsProdOutMax=[]  UintegralTsProdOutMin=[]  UintegralTsProdOutMax=[]  UngainTsProdOutMin=[]  UngainTsProdOutMax=[]  ClampingZeroOutDataTypeStr=Inherit: Inherit via back propagation  ClampingZeroOutMin=[]  ClampingZeroOutMax=[]  FilterDenConstantOutDataTypeStr=Inherit: Inherit via back propagation  FilterDenConstantOutMin=[]  FilterDenConstantOutMax=[]  PCopyOutDataTypeStr=Inherit: Inherit via back propagation  PCopyOutMin=[]  PCopyOutMax=[]  NCopyOutDataTypeStr=Inherit: Inherit via back propagation  NCopyOutMin=[]  NCopyOutMax=[]  IntegratorContinuousStateAttributes=''  IntegratorStateMustResolveToSignalObject=off  IntegratorRTWStateStorageClass=Auto  FilterContinuousStateAttributes=''  FilterStateMustResolveToSignalObject=off  FilterRTWStateStorageClass=Auto  ParallelPVariant=InternalParameters  IdealPVariant=Disabled  IVariant=InternalParameters  DVariant=Disabled  IntegratorVariant=Discrete  SatVariant=Disabled  AWVariant=Passthrough  PCopyVariant=Disabled  TRVariant=Disabled  FdbkBlocksVariant=Forward  IdealPFdbkVariant=Disabled  SatFdbkVariant=Disabled  DerivativeFilterVariant=Disabled  NVariant=Disabled  NCopyVariant=Disabled_SignalSpec  FilterICVariant=Disabled  IntegratorICVariant=InternalICs  ExternalResetVariant=Disabled  TRSumVariant=Passthrough  SumFdbkVariant=Disabled  SumVariant=Sum_PI  TsampFilterVariant=InternalTs  TsampNgainVariant=Passthrough  TsampIntegralVariant=Disabled_SignalSpec  ExternalSaturationOutDataTypeStr=Inherit: Same as second input
  PID Frequency : slpidlib/PID Controller  Controller=PI  Form=Parallel  TimeDomain=Discrete-time  UseExternalTs=off  SampleTime=2*Ts  IntegratorMethod=Forward Euler  FilterMethod=Forward Euler  ControllerParametersSource=internal  P=KP_fre_resynch  I=KI_fre_resynch  UseKiTs=off  D=0  N=100  UseFilter=on  TunerSelectOption=Frequency Response Based  InitialConditionSource=internal  InitialConditionForIntegrator=0  InitialConditionForFilter=0  DifferentiatorICPrevScaledInput=0  ExternalReset=none  TrackingMode=off  Kt=1  LimitOutput=off  SatLimitsSource=internal  UpperSaturationLimit=0.05  LowerSaturationLimit=-0.05  LinearizeAsGain=on  AntiWindupMode=clamping  Kb=1  LimitIntegrator=off  UpperIntegratorSaturationLimit=inf  LowerIntegratorSaturationLimit=-inf  POutMin=[]  POutMax=[]  IOutMin=[]  IOutMax=[]  DOutMin=[]  DOutMax=[]  NOutMin=[]  NOutMax=[]  SumOutMin=[]  SumOutMax=[]  SaturationOutMin=[]  SaturationOutMax=[]  PParamMin=[]  PParamMax=[]  IParamMin=[]  IParamMax=[]  DParamMin=[]  DParamMax=[]  NParamMin=[]  NParamMax=[]  KbParamMin=[]  KbParamMax=[]  KtParamMin=[]  KtParamMax=[]  KbOutMin=[]  KbOutMax=[]  KtOutMin=[]  KtOutMax=[]  IntegratorOutMin=[]  IntegratorOutMax=[]  FilterOutMin=[]  FilterOutMax=[]  SumI1OutMin=[]  SumI1OutMax=[]  SumI2OutMin=[]  SumI2OutMax=[]  SumI3OutMin=[]  SumI3OutMax=[]  SumI4OutMin=[]  SumI4OutMax=[]  SumDOutMin=[]  SumDOutMax=[]  DifferentiatorOutMin=[]  DifferentiatorOutMax=[]  FilterDiffOutCoefMin=[]  FilterDiffOutCoefMax=[]  ReciprocalOutMin=[]  ReciprocalOutMax=[]  SumDenOutMin=[]  SumDenOutMax=[]  SumNumOutMin=[]  SumNumOutMax=[]  DivideOutMin=[]  DivideOutMax=[]  UdiffTsProdOutMin=[]  UdiffTsProdOutMax=[]  NTsProdOutMin=[]  NTsProdOutMax=[]  UintegralTsProdOutMin=[]  UintegralTsProdOutMax=[]  UngainTsProdOutMin=[]  UngainTsProdOutMax=[]  ClampingZeroOutDataTypeStr=Inherit: Inherit via back propagation  ClampingZeroOutMin=[]  ClampingZeroOutMax=[]  FilterDenConstantOutDataTypeStr=Inherit: Inherit via back propagation  FilterDenConstantOutMin=[]  FilterDenConstantOutMax=[]  PCopyOutDataTypeStr=Inherit: Inherit via back propagation  PCopyOutMin=[]  PCopyOutMax=[]  NCopyOutDataTypeStr=Inherit: Inherit via back propagation  NCopyOutMin=[]  NCopyOutMax=[]  IntegratorContinuousStateAttributes=''  IntegratorStateMustResolveToSignalObject=off  IntegratorRTWStateStorageClass=Auto  FilterContinuousStateAttributes=''  FilterStateMustResolveToSignalObject=off  FilterRTWStateStorageClass=Auto  ParallelPVariant=InternalParameters  IdealPVariant=Disabled  IVariant=InternalParameters  DVariant=Disabled  IntegratorVariant=Discrete  SatVariant=Disabled  AWVariant=Passthrough  PCopyVariant=Disabled  TRVariant=Disabled  FdbkBlocksVariant=Forward  IdealPFdbkVariant=Disabled  SatFdbkVariant=Disabled  DerivativeFilterVariant=Disabled  NVariant=Disabled  NCopyVariant=Disabled_SignalSpec  FilterICVariant=Disabled  IntegratorICVariant=InternalICs  ExternalResetVariant=Disabled  TRSumVariant=Passthrough  SumFdbkVariant=Disabled  SumVariant=Sum_PI  TsampFilterVariant=InternalTs  TsampNgainVariant=Passthrough  TsampIntegralVariant=Disabled_SignalSpec  ExternalSaturationOutDataTypeStr=Inherit: Same as second input
  PID voltage : slpidlib/PID Controller  Controller=PI  Form=Parallel  TimeDomain=Discrete-time  UseExternalTs=off  SampleTime=2*Ts  IntegratorMethod=Forward Euler  FilterMethod=Forward Euler  ControllerParametersSource=internal  P=KP_Vol_resynch  I=KI_Vol_resynch  UseKiTs=off  D=0  N=100  UseFilter=on  TunerSelectOption=Frequency Response Based  InitialConditionSource=internal  InitialConditionForIntegrator=0.995  InitialConditionForFilter=0  DifferentiatorICPrevScaledInput=0  ExternalReset=none  TrackingMode=off  Kt=1  LimitOutput=off  SatLimitsSource=internal  UpperSaturationLimit=0.05  LowerSaturationLimit=-0.05  LinearizeAsGain=on  AntiWindupMode=clamping  Kb=1  LimitIntegrator=off  UpperIntegratorSaturationLimit=inf  LowerIntegratorSaturationLimit=-inf  POutMin=[]  POutMax=[]  IOutMin=[]  IOutMax=[]  DOutMin=[]  DOutMax=[]  NOutMin=[]  NOutMax=[]  SumOutMin=[]  SumOutMax=[]  SaturationOutMin=[]  SaturationOutMax=[]  PParamMin=[]  PParamMax=[]  IParamMin=[]  IParamMax=[]  DParamMin=[]  DParamMax=[]  NParamMin=[]  NParamMax=[]  KbParamMin=[]  KbParamMax=[]  KtParamMin=[]  KtParamMax=[]  KbOutMin=[]  KbOutMax=[]  KtOutMin=[]  KtOutMax=[]  IntegratorOutMin=[]  IntegratorOutMax=[]  FilterOutMin=[]  FilterOutMax=[]  SumI1OutMin=[]  SumI1OutMax=[]  SumI2OutMin=[]  SumI2OutMax=[]  SumI3OutMin=[]  SumI3OutMax=[]  SumI4OutMin=[]  SumI4OutMax=[]  SumDOutMin=[]  SumDOutMax=[]  DifferentiatorOutMin=[]  DifferentiatorOutMax=[]  FilterDiffOutCoefMin=[]  FilterDiffOutCoefMax=[]  ReciprocalOutMin=[]  ReciprocalOutMax=[]  SumDenOutMin=[]  SumDenOutMax=[]  SumNumOutMin=[]  SumNumOutMax=[]  DivideOutMin=[]  DivideOutMax=[]  UdiffTsProdOutMin=[]  UdiffTsProdOutMax=[]  NTsProdOutMin=[]  NTsProdOutMax=[]  UintegralTsProdOutMin=[]  UintegralTsProdOutMax=[]  UngainTsProdOutMin=[]  UngainTsProdOutMax=[]  ClampingZeroOutDataTypeStr=Inherit: Inherit via back propagation  ClampingZeroOutMin=[]  ClampingZeroOutMax=[]  FilterDenConstantOutDataTypeStr=Inherit: Inherit via back propagation  FilterDenConstantOutMin=[]  FilterDenConstantOutMax=[]  PCopyOutDataTypeStr=Inherit: Inherit via back propagation  PCopyOutMin=[]  PCopyOutMax=[]  NCopyOutDataTypeStr=Inherit: Inherit via back propagation  NCopyOutMin=[]  NCopyOutMax=[]  IntegratorContinuousStateAttributes=''  IntegratorStateMustResolveToSignalObject=off  IntegratorRTWStateStorageClass=Auto  FilterContinuousStateAttributes=''  FilterStateMustResolveToSignalObject=off  FilterRTWStateStorageClass=Auto  ParallelPVariant=InternalParameters  IdealPVariant=Disabled  IVariant=InternalParameters  DVariant=Disabled  IntegratorVariant=Discrete  SatVariant=Disabled  AWVariant=Passthrough  PCopyVariant=Disabled  TRVariant=Disabled  FdbkBlocksVariant=Forward  IdealPFdbkVariant=Disabled  SatFdbkVariant=Disabled  DerivativeFilterVariant=Disabled  NVariant=Disabled  NCopyVariant=Disabled_SignalSpec  FilterICVariant=Disabled  IntegratorICVariant=InternalICs  ExternalResetVariant=Disabled  TRSumVariant=Passthrough  SumFdbkVariant=Disabled  SumVariant=Sum_PI  TsampFilterVariant=InternalTs  TsampNgainVariant=Passthrough  TsampIntegralVariant=Disabled_SignalSpec  ExternalSaturationOutDataTypeStr=Inherit: Same as second input
  Product : Product
  Product1 : Product
  Product2 : Product
  Relational Operator : RelationalOperator  Operator=<=  OutDataTypeStr=boolean  RndMeth=Simplest  InputSameDT=off
  Relational Operator1 : RelationalOperator  Operator=<=  OutDataTypeStr=boolean  RndMeth=Simplest  InputSameDT=off
  Relational Operator2 : RelationalOperator  Operator=<=  OutDataTypeStr=boolean  RndMeth=Simplest  InputSameDT=off
  Resynchronization Time Delay : Subsystem
  Sum : Sum  Inputs=|+-
  Sum1 : Sum  Inputs=|+-
  Sum2 : Sum  Inputs=|+-
  Sum3 : Sum  Inputs=++|
  Synch Voltage : Subsystem
  pu1 : Gain  Gain=1/Grid.Frequency
  pu2 : Gain  Gain=1/Microgrid.radtodegree
  pu3 : Gain  Gain=1/Grid.Frequency
  pu4 : Gain  Gain=1/Microgrid.radtodegree
  Bus Element Out : Outport  PortName=MGController  Element=resynch
  Bus Element Out1 : Outport  PortName=MGController  Element=synchfrequency
  Bus Element Out2 : Outport  PortName=MGController  Element=synchvoltage
  Bus Element Out3 : Outport  PortName=MGController  Element=synchvoltagedpr
  Bus Element Out4 : Outport  PortName=MGController  Element=frequencyerror
  Bus Element Out5 : Outport  PortName=MGController  Element=phaseerror
  Bus Element Out6 : Outport  PortName=MGController  Element=voltagemagerror
  wires:
  Sum/1 -> Product1/1
  pu1/1 -> Sum/1
  pu4/1 -> Sum2/2
  pu2/1 -> Sum2/1
  pu3/1 -> Sum/2
  In Bus Element2/1 -> pu4/1
  In Bus Element3/1 -> pu3/1
  Sum1/1 -> Product2/1
  Constant/1 -> Relational Operator/2
  Constant1/1 -> Relational Operator1/2
  Constant2/1 -> Relational Operator2/2
  Relational Operator/1 -> Logical Operator/1
  Relational Operator1/1 -> Logical Operator/2
  Relational Operator2/1 -> Logical Operator/3
  Sum3/1 -> Bus Element Out1/1
  PID Frequency/1 -> Sum3/1
  PID Angle/1 -> Sum3/2
  Sum2/1 -> Product/1
  Product/1 -> Bus Element Out5/1, PID Angle/1, Relational Operator1/1
  Product1/1 -> Relational Operator/1, Bus Element Out4/1, PID Frequency/1
  Product2/1 -> Relational Operator2/1, PID voltage/1, Bus Element Out6/1
  Bus Element In/1 -> Product1/2
  Bus Element In1/1 -> Product/2
  Bus Element In2/1 -> Product2/2
  In Bus Element7/1 -> pu1/1
  In Bus Element1/1 -> pu2/1
  In Bus Element4/1 -> Sum1/1
  In Bus Element5/1 -> Sum1/2
  PID voltage/1 -> Synch Voltage/1(MicrogridController), Bus Element Out2/1
  Bus Element In3/1 -> Resynchronization Time Delay/2(ResynchronizationCmd)
  Resynchronization Time Delay/1(MGController) -> [Resynch], Bus Element Out/1
  Logical Operator/1 -> Resynchronization Time Delay/1(Resynchronization)
  Bus Element In4/1 -> Synch Voltage/2(ControlRoom)
  Bus Element In5/1 -> Synch Voltage/3(ReactivePower)
  Synch Voltage/1(SynchVoltage) -> Bus Element Out3/1
  [Resynch] -> Synch Voltage/4(Resynch)

== system remoteMicrogrid/Operator Control Room/Measurements and visualizations /BESS, PV and Load Measurements/Active and reactive Power ==
  Grid Active Power : Inport
  BESS Active Power : Inport  Port=2
  Load Active Power : Inport  Port=3
  PV Active Power : Inport  Port=4
  Grid Reactive Power : Inport  Port=5
  BESS Reactive Power : Inport  Port=6
  Load Reactive Power : Inport  Port=7
  Bus Creator : BusCreator  Inputs=4
  Bus Creator1 : BusCreator  Inputs=3
  Power  Measurements : Scope  NumInputPorts=2
  Active Power : Outport
  ReActive Power : Outport  Port=2
  wires:
  BESS Active Power/1 -> Bus Creator/2
  BESS Reactive Power/1 -> Bus Creator1/2
  Bus Creator1/1 -> ReActive Power/1, Power  Measurements/2
  Bus Creator/1 -> Active Power/1, Power  Measurements/1
  Grid Active Power/1 -> Bus Creator/1
  PV Active Power/1 -> Bus Creator/4
  Load Active Power/1 -> Bus Creator/3
  Grid Reactive Power/1 -> Bus Creator1/1
  Load Reactive Power/1 -> Bus Creator1/3

== system remoteMicrogrid/Operator Control Room/Measurements and visualizations /BESS, PV and Load Measurements/BESS and PV Measurements ==
  Vpv (V) : Inport
  Vabc : Inport  Port=2
  Iabc : Inport  Port=3
  Ipv (A) : Inport  Port=4
  Vpvac : Inport  Port=5
  Ipvac : Inport  Port=6
  PV Active Power : Inport  Port=7
  BESS Measurements : Scope  NumInputPorts=4
  Gain : Gain  Gain=0.1
  Iabc1 : InportShadow  Port=3
  "Inverter Active & Reactive Power " : Subsystem
  Mux1 : Mux  Inputs=2
  PV Measurmeents : Scope  NumInputPorts=4
  Vabc1 : InportShadow  Port=2
  wires:
  Vpv (V)/1 -> PV Measurmeents/1  "PV Voltage (V)"
  PV Active Power/1 -> PV Measurmeents/3  "PV Power (kW)"
  "Inverter Active & Reactive Power "/2(Q) -> BESS Measurements/2  "BESS  Reactive Power (pu)"
  Vabc1/1 -> BESS Measurements/3  "BESS Voltage (pu)"
  Mux1/1 -> PV Measurmeents/4  "AC voltage/10 (V) and current (A)"
  Gain/1 -> Mux1/1  "Vac/10"
  Ipv (A)/1 -> PV Measurmeents/2  "PV Current (A)"
  "Inverter Active & Reactive Power "/1(P) -> BESS Measurements/1  "BESS  Active Power (pu)"
  Iabc/1 -> "Inverter Active & Reactive Power "/2(Iabc)  "BESS Current (pu)"
  Vabc/1 -> "Inverter Active & Reactive Power "/1(Vabc)  "BESS Voltage (pu)"
  Iabc1/1 -> BESS Measurements/4  "BESS Current (pu)"
  Vpvac/1 -> Gain/1
  Ipvac/1 -> Mux1/2

== system remoteMicrogrid/Operator Control Room/Measurements and visualizations /BESS, PV and Load Measurements/Load 1 Measurements ==
  Load Active Power : Inport
  Load Reactive Power : Inport  Port=2
  Load Current(p.u.) : Inport  Port=3
  Load Voltage (p.u.) : Inport  Port=4
  Load Voltage RMS (p.u.) : Inport  Port=5
  Bus Creator4 : BusCreator  Inputs=2
  Load Measurements : Scope  NumInputPorts=4
  wires:
  Load Current(p.u.)/1 -> Load Measurements/2  "Load Current(p.u.)"
  Bus Creator4/1 -> Load Measurements/1  "Load Active Power (kW) and reactive power (KVAr)"
  Load Reactive Power/1 -> Bus Creator4/2  "Load Reactive Power (KVAr)"
  Load Voltage RMS (p.u.)/1 -> Load Measurements/4  "Load Voltage RMS (p.u.)"
  Load Active Power/1 -> Bus Creator4/1  "Load Active Power (KW)"
  Load Voltage (p.u.)/1 -> Load Measurements/3  "Load Voltage (p.u.)"

== system remoteMicrogrid/Operator Control Room/Measurements and visualizations /BESS, PV and Load Measurements/Load 1 Measurements1 ==
  Load Active Power : Inport
  Load Reactive Power : Inport  Port=2
  Load Current(p.u.) : Inport  Port=3
  Load Voltage (p.u.) : Inport  Port=4
  Load Voltage RMS (p.u.) : Inport  Port=5
  Bus Creator4 : BusCreator  Inputs=2
  Load Measurements : Scope  NumInputPorts=4
  wires:
  Load Voltage (p.u.)/1 -> Load Measurements/3  "Load Voltage (p.u.)"
  Load Active Power/1 -> Bus Creator4/1  "Load Active Power (KW)"
  Load Voltage RMS (p.u.)/1 -> Load Measurements/4  "Load Voltage RMS (p.u.)"
  Load Reactive Power/1 -> Bus Creator4/2  "Load Reactive Power (KVAr)"
  Bus Creator4/1 -> Load Measurements/1  "Load Active Power (kW) and reactive power (KVAr)"
  Load Current(p.u.)/1 -> Load Measurements/2  "Load Current(p.u.)"
